simulink library "INT_RailP_PRV"  (R2016b)
settings: Solver=VariableStepAuto  StartTime=0.0  StopTime=10.0  RelTol=1e-3
settings Model: Creator=shiliwei  LastModifiedBy=shiliwei

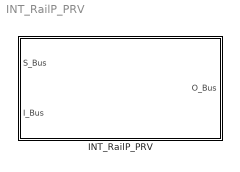
== system INT_RailP_PRV ==
  INT_RailP_PRV : Subsystem

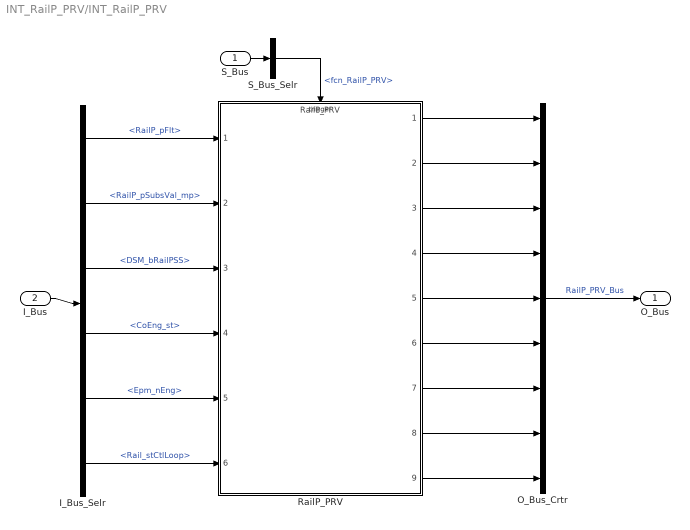
== system INT_RailP_PRV/INT_RailP_PRV ==
  S_Bus : Inport
  I_Bus : Inport  Port=2
  I_Bus_Selr : BusSelector  OutputSignals=RailP_pFlt,RailP_pSubsVal_mp,DSM_bRailPSS,CoEng_st,Epm_nEng,Rail_stCtlLoop
  O_Bus_Crtr : BusCreator  Inputs=9
  RailP_PRV : ModelReference  ModelNameDialog=RailP_PRV  SimulationMode=Normal  ModelReferenceVersion=1.208  TriggerPortName=function  TriggerPortTriggerType=function-call  TriggerPortStatesWhenEnabling=held
  S_Bus_Selr : BusSelector  OutputSignals=fcn_RailP_PRV
  O_Bus : Outport
  wires:
  S_Bus_Selr/1 -> RailP_PRV/Trigger  "<fcn_RailP_PRV>"
  S_Bus/1 -> S_Bus_Selr/1
  I_Bus/1 -> I_Bus_Selr/1
  I_Bus_Selr/1 -> RailP_PRV/1  "<RailP_pFlt>"
  I_Bus_Selr/2 -> RailP_PRV/2  "<RailP_pSubsVal_mp>"
  I_Bus_Selr/3 -> RailP_PRV/3  "<DSM_bRailPSS>"
  I_Bus_Selr/4 -> RailP_PRV/4  "<CoEng_st>"
  I_Bus_Selr/5 -> RailP_PRV/5  "<Epm_nEng>"
  I_Bus_Selr/6 -> RailP_PRV/6  "<Rail_stCtlLoop>"
  O_Bus_Crtr/1 -> O_Bus/1  "RailP_PRV_Bus"
  RailP_PRV/1 -> O_Bus_Crtr/1
  RailP_PRV/2 -> O_Bus_Crtr/2
  RailP_PRV/3 -> O_Bus_Crtr/3
  RailP_PRV/4 -> O_Bus_Crtr/4
  RailP_PRV/5 -> O_Bus_Crtr/5
  RailP_PRV/6 -> O_Bus_Crtr/6
  RailP_PRV/7 -> O_Bus_Crtr/7
  RailP_PRV/8 -> O_Bus_Crtr/8
  RailP_PRV/9 -> O_Bus_Crtr/9
